simulink model "vdp_Local2"  (R2021a)
settings: Solver=VariableStepAuto  StartTime=0.0  StopTime=10.0  RelTol=1e-3
settings Model: Creator=20204920  LastModifiedBy=20204920

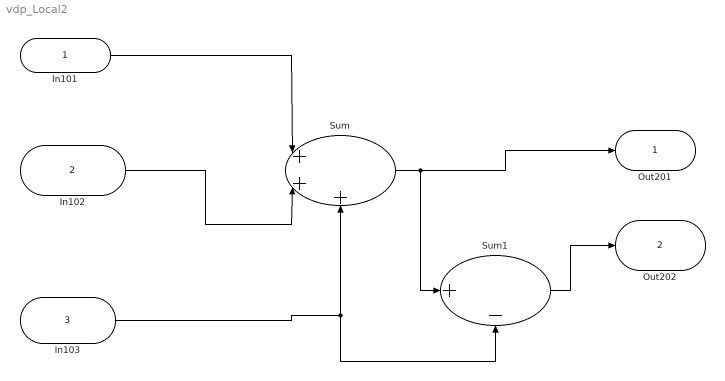
== system vdp_Local2 ==
  In101 : Inport
  In102 : Inport  Port=2
  In103 : Inport  Port=3
  Sum : Sum  Inputs=|+++
  Sum1 : Sum  Inputs=|+-
  Out201 : Outport
  Out202 : Outport  Port=2
  wires:
  In101/1 -> Sum/1
  In102/1 -> Sum/2
  In103/1 -> Sum1/2, Sum/3
  Sum/1 -> Sum1/1, Out201/1
  Sum1/1 -> Out202/1
